simulink model "source_filter"  (R2016b)
settings: Solver=VariableStepAuto  StartTime=0.0  StopTime=10.0  RelTol=1e-3
libraries: fl_lib x11
settings Model: Creator=WANGSP1  LastModifiedBy=WANGSP1

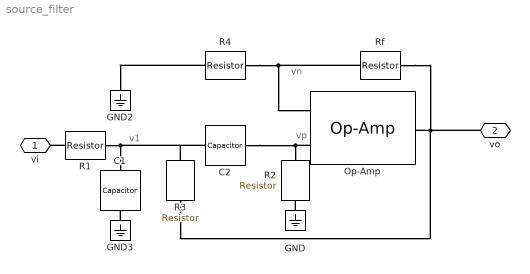
== system source_filter ==
  note: v1
  note: vp
  note: vn
  C1 : fl_lib/Electrical/Electrical Elements/Capacitor  c=1e-6 F  r=1e-6 Ohm  g=0 1/Ohm  i_specify=off  i_priority=None  i=0 A  v_specify=off  v_priority=None  v=0 V  vc_specify=on  vc_priority=None  vc=0 V
  C2 : fl_lib/Electrical/Electrical Elements/Capacitor  c=1e-6 F  r=1e-6 Ohm  g=0 1/Ohm  i_specify=off  i_priority=None  i=0 A  v_specify=off  v_priority=None  v=0 V  vc_specify=on  vc_priority=None  vc=0 V
  GND : fl_lib/Electrical/Electrical Elements/Electrical Reference
  GND2 : fl_lib/Electrical/Electrical Elements/Electrical Reference
  GND3 : fl_lib/Electrical/Electrical Elements/Electrical Reference
  Op-Amp : fl_lib/Electrical/Electrical Elements/Op-Amp  outI_specify=off  outI_priority=None  outI=0 A
  R{1..4} (4 alike) : fl_lib/Electrical/Electrical Elements/Resistor  R=1 Ohm  i_specify=off  i_priority=None  i=0 A  v_specify=off  v_priority=None  v=0 V
  Rf : fl_lib/Electrical/Electrical Elements/Resistor  R=1 Ohm  i_specify=off  i_priority=None  i=0 A  v_specify=off  v_priority=None  v=0 V
  vi : PMIOPort  Port=1  Side=Left
  vo : PMIOPort  Port=2  Side=Right
  connections:
  R4/LConn1 -- GND2/LConn1
  R4/RConn1 -- Rf/LConn1 -- Op-Amp/LConn2
  Rf/RConn1 -- vo/RConn1 -- R3/RConn1 -- Op-Amp/RConn1
  R1/RConn1 -- C2/LConn1 -- R3/LConn1 -- C1/LConn1
  Op-Amp/LConn1 -- C2/RConn1 -- R2/LConn1
  GND/LConn1 -- R2/RConn1
  GND3/LConn1 -- C1/RConn1
  R1/LConn1 -- vi/RConn1
